simulink model "problem_4"  (R2020b)
settings: Solver=VariableStepAuto  StartTime=0.0  StopTime=10.0  RelTol=1e-3
PreLoadFcn:
  | vars
values from neighbouring files (symbols this model uses):
  b = 0.1    [vars.m]
  J = 0.0100    (= 0.01)    [vars.m]
  k = 0.0100    (= 0.01)    [vars.m]
  L = 0.5    [vars.m]
  r = 1    [vars.m]
settings Model: Creator=hp  LastModifiedBy=hp

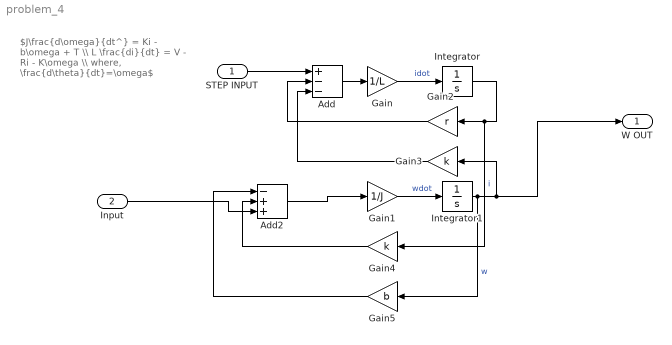
== system problem_4 ==
  note: $J\frac{d\omega}{dt^} = Ki - b\omega + T \\ L \frac{di}{dt} = V - Ri - K\omega \\ where, \frac{d\theta}{dt}=\omega$
  STEP INPUT : Inport
  Input : Inport  Port=2
  Add : Sum  Inputs=+--
  Add2 : Sum  Inputs=-++
  Gain : Gain  Gain=1/L
  Gain1 : Gain  Gain=1/J
  Gain2 : Gain  Gain=r
  Gain3 : Gain  Gain=k
  Gain4 : Gain  Gain=k
  Gain5 : Gain  Gain=b
  Integrator : Integrator
  Integrator1 : Integrator
  W OUT : Outport
  wires:
  Input/1 -> Add2/3
  Gain4/1 -> Add2/2
  Gain1/1 -> Integrator1/1  "wdot"
  Gain5/1 -> Add2/1
  Integrator1/1 -> Gain5/1, W OUT/1, Gain3/1  "w"
  Gain/1 -> Integrator/1  "idot"
  Gain2/1 -> Add/2
  Add/1 -> Gain/1
  STEP INPUT/1 -> Add/1
  Gain3/1 -> Add/3
  Integrator/1 -> Gain2/1, Gain4/1  "i"
  Add2/1 -> Gain1/1
